simulink model "schaltwerk_zaehler"  (R2024a)
settings: Solver=ode45  StartTime=0.0  StopTime=inf  RelTol=1e-3  EnableMultiTasking=on
libraries: simulink_extras x2
settings Model: Creator=nunkesser  LastModifiedBy=nunkesser
settings SolverCC: AlgebraicLoopSolver=TrustRegion
settings DataIOCC: LimitDataPoints=on  SaveFormat=Array  ReturnWorkspaceOutputs=off
settings OptimizationCC: LifeSpan=inf
settings DebuggingCC: SolverPrmCheckMsg=warning  UnconnectedInputMsg=warning  UnconnectedOutputMsg=warning  UnconnectedLineMsg=warning  AllowSymbolicDim=off  SFUnexpectedBacktrackingDiag=warning  SFNoUnconditionalDefaultTransitionDiag=warning  SFExecutionAtInitializationDiag=none  ArithmeticOperatorsInVariantConditions=warning
settings HardwareCC: ProdBitPerPointer=32  ProdBitPerSizeT=32  ProdBitPerPtrDiffT=32  ProdLargestAtomicFloat=None  ProdIntDivRoundTo=Undefined  ProdEndianess=Unspecified  ProdWordSize=32  ProdHWDeviceType=32-bit Generic
settings ModelReferenceCC: EnableRefExpFcnMdlSchedulingChecks=on  PropagateSignalLabelsOutOfModel=off
settings SFSimCC: SimUseLocalCustomCode=off  CustomCodeUndefinedFunction=UseInterfaceOnly
settings RTWCC: RTWUseLocalCustomCode=off  GPUComputeCapability=3.5
settings CodeAppCC: StateflowObjectComments=on
settings GRTTargetCC: TargetLangStandard=C89/C90 (ANSI)
settings ConfigComp: CovMetricSettings=dw  CovSaveCumulativeToWorkspaceVar=on  CovSaveSingleToWorkspaceVar=on  CovExternalEMLEnable=off  CovSFcnEnable=off

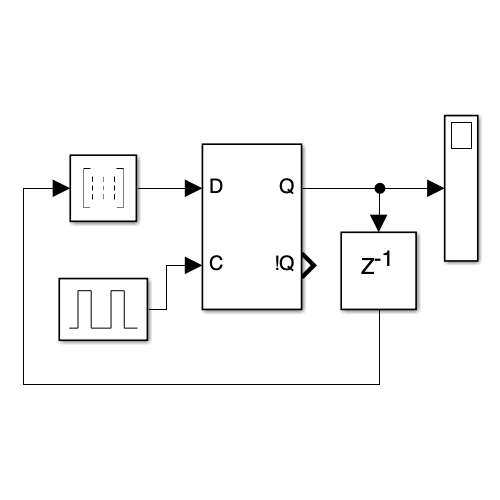
[thumbnail: Simulink's stored preview of the top-level diagram]
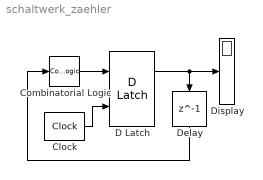
== system schaltwerk_zaehler ==
  Clock : simulink_extras/Flip Flops/Clock  period=2
  Combinatorial Logic : CombinatorialLogic  TruthTable=|
      | [
      | 0 0 0 1;0 0 1 0;
      | 0 0 1 1;0 1 0 0;
      | 0 1 0 1;0 1 1 0;
      | 0 1 1 1;1 0 0 0;
      | 1 0 0 1;1 0 1 0;
      | 1 0 1 1;1 1 0 0;
      | 1 1 0 1;1 1 1 0;
      | 1 1 1 1;0 0 0 0
      | ]
  D Latch : simulink_extras/Flip Flops/D Latch
  Delay : Delay  DelayLength=1  InitialCondition=0
  Display : Display
  wires:
  Combinatorial Logic/1 -> D Latch/1
  D Latch/1 -> Display/1, Delay/1
  Clock/1 -> D Latch/2
  Delay/1 -> Combinatorial Logic/1
